simulink model "Grid_Connected_Solar_PV_Array"  (R2023b)
settings: Solver=VariableStepAuto  StartTime=0.0  StopTime=0.5  RelTol=1e-3
undefined symbols (not defined in the file): Ts_Control, Ts_Power
libraries: spsSeriesRLCBranchLib x5, slpidlib x2, spsVoltageMeasurementLib x2, spsACVoltageSourceLib x1, spsCurrentMeasurementLib x1, spsPVArrayLib x1, spsPWMGenerator2LevelLib x1, spsSeriesRLCLoadLib x1, spsFundamentalPLLDrivenLib x1, spsMeanLib x1, spsPLLLib x1, spsAlphaBetaZerotodq0Lib x1
settings Model: Creator=HP  LastModifiedBy=HP
settings DataIOCC: SaveOutput=off  SaveState=on  SignalLogging=off  DSMLogging=off  ReturnWorkspaceOutputs=off  LoggingToFile=on

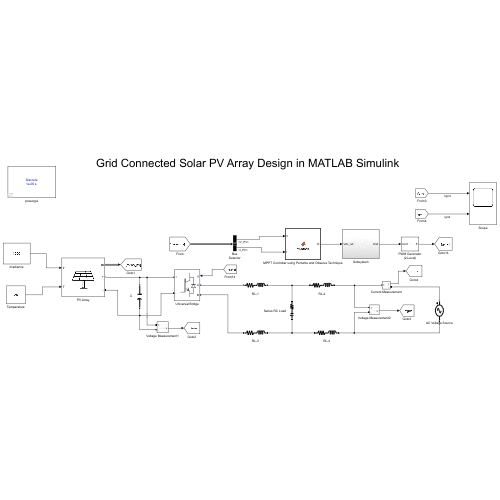
[thumbnail: Simulink's stored preview of the top-level diagram]
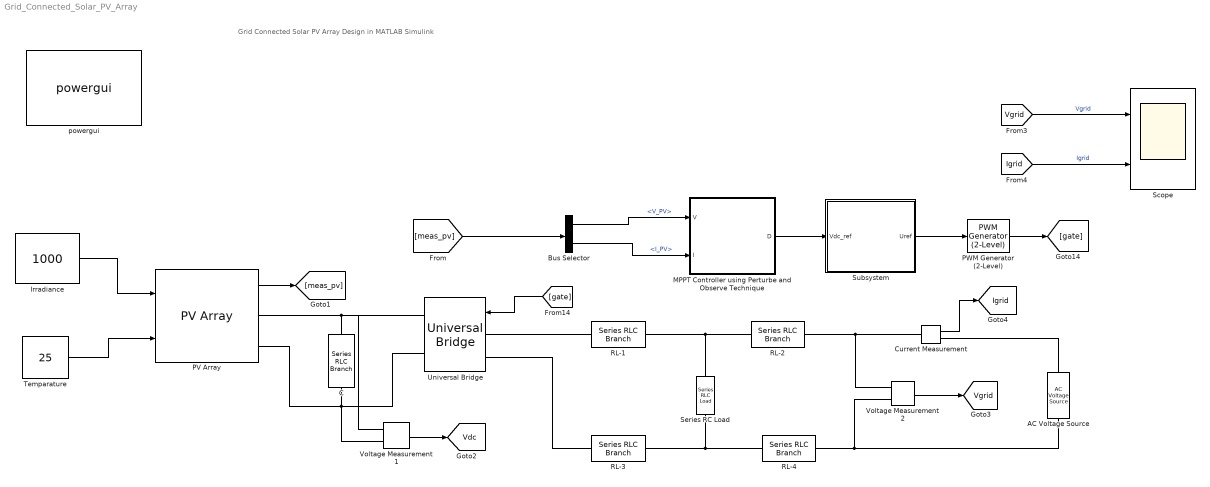
== system Grid_Connected_Solar_PV_Array ==
  note: Grid Connected Solar PV Array Design in MATLAB Simulink
  AC Voltage Source : spsACVoltageSourceLib/AC Voltage Source  Amplitude=240*sqrt(2)  Phase=0  Frequency=50  SampleTime=0  Measurements=None  BusType=swing  Pref=10e3  Qref=0  Qmin=-inf  Qmax=+inf
  Bus Selector : BusSelector  OutputSignals=V_PV,I_PV
  C : spsSeriesRLCBranchLib/Series RLC Branch  LConnTagsString=__new0  RConnTagsString=__new0  BranchType=C  Resistance=1  Inductance=1e-3  SetiL0=off  InitialCurrent=0  Capacitance=3000e-6  Setx0=on  InitialVoltage=420  Measurements=None
  Current Measurement : spsCurrentMeasurementLib/Current Measurement  PhasorSimulation=off  OutputType=Complex  PSBequivalent=0
  Irradiance : Constant  Value=1000
  MPPT Controller using Perturbe and Observe Technique : MATLAB Function  TreatAsAtomicUnit=on
  PV Array : spsPVArrayLib/PV Array  Npar=1  Nser=14  PlotType=array @ 1000 W/m2 & specified temperatures  S_vec="[ 1000  500  100 ]"  Temp_C_vec="[ 45 25  ]"  ModuleName=A10Green Technology A10J-M60-240  PlotWhenSelected=off  Pm=240.5376  Ncell=60  Voc=36.84  Isc=8.32  Vm=30.72  Im=7.83  beta_Voc_pc=-0.359  alpha_Isc_pc=0.096995  beta_Voc=-0.13226  alpha_Isc=0.00807  IL=8.3299  I0=2.8736e-10  nI=0.99259  Rsh=330.6558  Rs=0.19366  RobustModel=off  RobustCellTemperature=313.3991  BAL=on  Tc=1e-6  Tfilter=5e-5
  PWM Generator (2-Level) : spsPWMGenerator2LevelLib/PWM Generator (2-Level)  ModulatorType=Single-phase full-bridge (4 pulses)  ModulatorMode=Unsynchronized  Fc=5e3  Pc=90  nF=27  MinMax="[ -1  1 ]"  SamplingTechnique=Natural  ModulatingSignals=off  m=0.8  Freq=60  Phase=0  Ts=Ts_Power  ShowCarrierOutport=off
  RL-{1..4} (4 alike) : spsSeriesRLCBranchLib/Series RLC Branch  LConnTagsString=__new0  RConnTagsString=__new0  BranchType=RL  Resistance=8.2e-3  Inductance=2.18e-3  SetiL0=off  InitialCurrent=0  Capacitance=3000e-6  Setx0=on  InitialVoltage=420  Measurements=None
  Scope : Scope  NumInputPorts=2
  Series RC Load : spsSeriesRLCLoadLib/Series RLC Load  LConnTagsString=a  RConnTagsString=__new0  NominalVoltage=240  NominalFrequency=60  ActivePower=10  InductivePower=0  CapacitivePower=500  Setx0=off  InitialVoltage=0  SetiL0=off  InitialCurrent=0  Measurements=None  LoadType=constant Z
  Subsystem : Subsystem
  Temparature : Constant  Value=25
  Universal Bridge : spsUniversalBridgeLib/Universal Bridge  Arms=2  SnubberResistance=1e5  SnubberCapacitance=inf  Device=IGBT / Diodes  Ron=1e-3  Lon=0  ForwardVoltages="[  0  0  ]"  ForwardVoltage=0  GTOparameters=[ 10e-6 , 20e-6 ]  IGBTparameters=[ 1e-6 , 2e-6 ]  Measurements=None  Measurements_2=None  converterType=Rectifier
  Voltage Measurement1 : spsVoltageMeasurementLib/Voltage Measurement  PhasorSimulation=off  OutputType=Complex  PSBequivalent=0
  Voltage Measurement2 : spsVoltageMeasurementLib/Voltage Measurement  PhasorSimulation=off  OutputType=Complex  PSBequivalent=0
  powergui : sps_lib/powergui  Priority=1  SimulationMode=Discrete  SampleTime=Ts_Power  frequency=60  Iterations=50  frequencyindice=50  Pbase=100e6  ErrMax=1e-4  UnitsV=kV  UnitsW=MW  buscounter=0  FunctionMessages=off  echomessages=off  EnableUseOfTLC=off  CurrentSourceSwitches=off  DisableSnubberDevices=off  DisableRonSwitches=off  DisableVfSwitches=off  DisplayEquations=off  AutomaticDiscreteSolvers=off  SolverType=Tustin/Backward Euler (TBE)  Interpol=off  ExternalGateDelay=off  methode=off  Ts=100  x0status=blocks  SPID=on  SwTol=0  HookPort=off  NonlinearTolerance=1e-4  nMaxIteration=100  ContinueOnMaxIteration=off  RestoreLinks=warning  ResistiveCurrentMeasurement=off  Frange=[0:2:500]  Ylog=off  Xlog=on  ShowGrid=off  save=off  variable=ZData  structure=0  ZoomFFT=off  StartTime=0.0  cycles=1  DisplayStyle=1  fundamental=60  FreqAxis=off  MaxFrequency=1000  frequencyindicesteady=1  RmsSteady=1  display=off
  tag scope: Igrid=global, Vdc=global, Vgrid=global
  wires:
  Temparature/1 -> PV Array/2
  PV Array/1 -> [meas_pv]
  Voltage Measurement1/1 -> [Vdc]
  Voltage Measurement2/1 -> [Vgrid]
  Current Measurement/1 -> [Igrid]
  [meas_pv] -> Bus Selector/1
  Bus Selector/1 -> MPPT Controller using Perturbe and Observe Technique/1(V)  "<V_PV>"
  Bus Selector/2 -> MPPT Controller using Perturbe and Observe Technique/2(I)  "<I_PV>"
  MPPT Controller using Perturbe and Observe Technique/1(D) -> Subsystem/1(Vdc_ref)
  Subsystem/1(Uref) -> PWM Generator (2-Level)/1
  PWM Generator (2-Level)/1 -> [gate]
  [gate] -> Universal Bridge/1
  [Vgrid] -> Scope/1  "Vgrid"
  [Igrid] -> Scope/2  "Igrid"
  Irradiance/1 -> PV Array/1
  connections:
  PV Array/RConn1 -- Universal Bridge/RConn1 -- Voltage Measurement1/LConn1 -- C/LConn1
  PV Array/RConn2 -- C/RConn1 -- Universal Bridge/RConn2 -- Voltage Measurement1/LConn2
  Universal Bridge/LConn1 -- RL-1/LConn1
  RL-3/LConn1 -- Universal Bridge/LConn2
  RL-2/LConn1 -- Series RC Load/LConn1 -- RL-1/RConn1
  RL-3/RConn1 -- RL-4/LConn1 -- Series RC Load/RConn1
  RL-2/RConn1 -- Current Measurement/LConn1 -- Voltage Measurement2/LConn1
  RL-4/RConn1 -- AC Voltage Source/LConn1 -- Voltage Measurement2/LConn2
  AC Voltage Source/RConn1 -- Current Measurement/RConn1

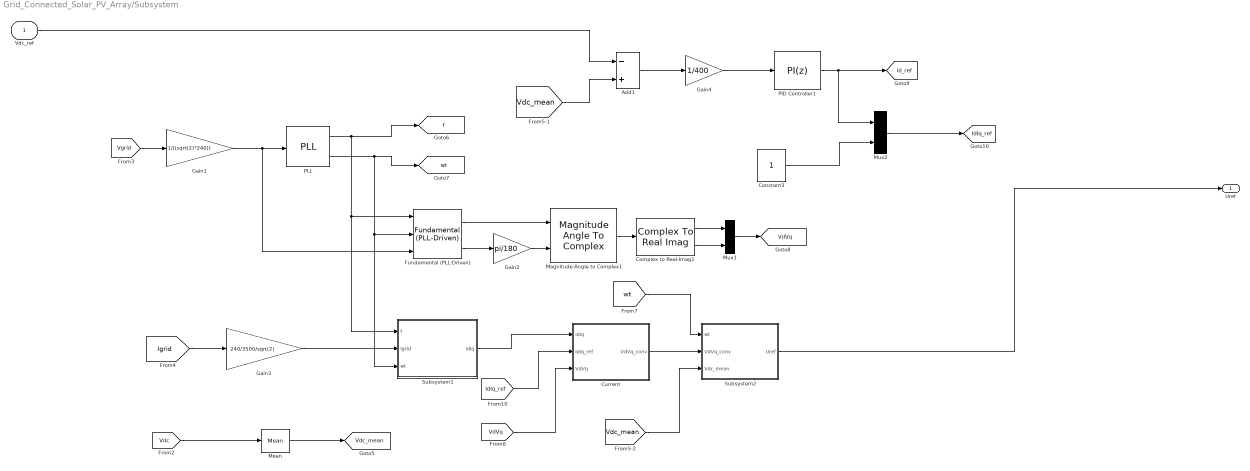
== system Grid_Connected_Solar_PV_Array/Subsystem ==
  Vdc_ref : Inport
  Add1 : Sum  Inputs=-+
  Complex to Real-Imag1 : ComplexToRealImag
  Constant3 : Constant
  Current : Subsystem
  Fundamental (PLL-Driven) : spsFundamentalPLLDrivenLib/Fundamental (PLL-Driven)  Finit=60  Fmin=45  InInit=[1, 0]  Ts=Ts_Control
      settings: LibrarySourceBlock=|
      | sps_lib/Sensors and Measurements/Fundamental
      | (PLL-Driven)
  Gain1 : Gain  Gain=1/((sqrt(2)*240))
  Gain2 : Gain  Gain=pi/180
  Gain3 : Gain  Gain=240/3500/sqrt(2)
  Gain4 : Gain  Gain=1/400
  Magnitude-Angle to Complex1 : MagnitudeAngleToComplex
  Mean : spsMeanLib/Mean  Freq=60  Vinit=420  Ts=Ts_Power
  Mux1 : Mux  Inputs=2
  Mux2 : Mux  Inputs=2
  PID Controller1 : slpidlib/PID Controller  Controller=PI  Form=Parallel  TimeDomain=Discrete-time  UseExternalTs=off  SampleTime=Ts_Control  IntegratorMethod=Forward Euler  FilterMethod=Forward Euler  ControllerParametersSource=internal  P=12  I=200  UseKiTs=off  D=0  N=100  UseFilter=on  TunerSelectOption=Transfer Function Based (PID Tuner App)  InitialConditionSource=internal  InitialConditionForIntegrator=0  InitialConditionForFilter=0  DifferentiatorICPrevScaledInput=0  ExternalReset=none  TrackingMode=off  Kt=1  LimitOutput=off  SatLimitsSource=internal  UpperSaturationLimit=inf  LowerSaturationLimit=-inf  LinearizeAsGain=on  AntiWindupMode=none  Kb=1  LimitIntegrator=off  UpperIntegratorSaturationLimit=inf  LowerIntegratorSaturationLimit=-inf  POutMin=[]  POutMax=[]  IOutMin=[]  IOutMax=[]  DOutMin=[]  DOutMax=[]  NOutMin=[]  NOutMax=[]  SumOutMin=[]  SumOutMax=[]  SaturationOutMin=[]  SaturationOutMax=[]  PParamMin=[]  PParamMax=[]  IParamMin=[]  IParamMax=[]  DParamMin=[]  DParamMax=[]  NParamMin=[]  NParamMax=[]  KbParamMin=[]  KbParamMax=[]  KtParamMin=[]  KtParamMax=[]  KbOutMin=[]  KbOutMax=[]  KtOutMin=[]  KtOutMax=[]  IntegratorOutMin=[]  IntegratorOutMax=[]  FilterOutMin=[]  FilterOutMax=[]  SumI1OutMin=[]  SumI1OutMax=[]  SumI2OutMin=[]  SumI2OutMax=[]  SumI3OutMin=[]  SumI3OutMax=[]  SumI4OutMin=[]  SumI4OutMax=[]  SumDOutMin=[]  SumDOutMax=[]  DifferentiatorOutMin=[]  DifferentiatorOutMax=[]  FilterDiffOutCoefMin=[]  FilterDiffOutCoefMax=[]  ReciprocalOutMin=[]  ReciprocalOutMax=[]  SumDenOutMin=[]  SumDenOutMax=[]  SumNumOutMin=[]  SumNumOutMax=[]  DivideOutMin=[]  DivideOutMax=[]  UdiffTsProdOutMin=[]  UdiffTsProdOutMax=[]  NTsProdOutMin=[]  NTsProdOutMax=[]  UintegralTsProdOutMin=[]  UintegralTsProdOutMax=[]  UngainTsProdOutMin=[]  UngainTsProdOutMax=[]  ClampingZeroOutDataTypeStr=Inherit: Inherit via back propagation  ClampingZeroOutMin=[]  ClampingZeroOutMax=[]  FilterDenConstantOutDataTypeStr=Inherit: Inherit via back propagation  FilterDenConstantOutMin=[]  FilterDenConstantOutMax=[]  PCopyOutDataTypeStr=Inherit: Inherit via back propagation  PCopyOutMin=[]  PCopyOutMax=[]  NCopyOutDataTypeStr=Inherit: Inherit via back propagation  NCopyOutMin=[]  NCopyOutMax=[]  IntegratorContinuousStateAttributes=''  IntegratorStateMustResolveToSignalObject=off  IntegratorRTWStateStorageClass=Auto  FilterContinuousStateAttributes=''  FilterStateMustResolveToSignalObject=off  FilterRTWStateStorageClass=Auto  ParallelPVariant=InternalParameters  IdealPVariant=Disabled  IVariant=InternalParameters  DVariant=Disabled  IntegratorVariant=Discrete  SatVariant=Disabled  AWVariant=Passthrough  PCopyVariant=Disabled  TRVariant=Disabled  FdbkBlocksVariant=Forward  IdealPFdbkVariant=Disabled  SatFdbkVariant=Disabled  DerivativeFilterVariant=Disabled  NVariant=Disabled  NCopyVariant=Disabled_SignalSpec  FilterICVariant=Disabled  IntegratorICVariant=InternalICs  ExternalResetVariant=Disabled  TRSumVariant=Passthrough  SumFdbkVariant=Disabled  SumVariant=Sum_PI  TsampFilterVariant=InternalTs  TsampNgainVariant=Passthrough  TsampIntegralVariant=Disabled_SignalSpec  ExternalSaturationOutDataTypeStr=Inherit: Same as second input
  PLL : spsPLLLib/PLL  Fmin=45  Par_Init=[0, 60]  ParK=[180, 3200, 1]  TcD=1e-4  MaxRateChangeFreq=12  FilterCutOffFreq=25  Ts=0  AGC=on
      settings: LibrarySourceBlock=sps_lib/Control/PLL
  Subsystem1 : Subsystem
  Subsystem2 : Subsystem
  Uref : Outport
  tag scope: IdIq_ref=global, Id_ref=global, VdVq=global, Vdc_mean=global, f=global, wt=global
  wires:
  [Vdc] -> Mean/1
  Mean/1 -> [Vdc_mean]
  Gain1/1 -> PLL/1, Fundamental (PLL-Driven)/3
  [Vgrid] -> Gain1/1
  PLL/1 -> Fundamental (PLL-Driven)/1, Subsystem1/1(f), [f]
  PLL/2 -> [wt], Fundamental (PLL-Driven)/2, Subsystem1/3(wt)
  Fundamental (PLL-Driven)/2 -> Gain2/1
  Fundamental (PLL-Driven)/1 -> Magnitude-Angle to Complex1/1
  Gain2/1 -> Magnitude-Angle to Complex1/2
  Magnitude-Angle to Complex1/1 -> Complex to Real-Imag1/1
  Complex to Real-Imag1/1 -> Mux1/1
  Complex to Real-Imag1/2 -> Mux1/2
  Mux1/1 -> [VdVq]
  [Igrid] -> Gain3/1
  Gain3/1 -> Subsystem1/2(Igrid)
  Vdc_ref/1 -> Add1/1
  [Vdc_mean] -> Add1/2
  Add1/1 -> Gain4/1
  Gain4/1 -> PID Controller1/1
  PID Controller1/1 -> Mux2/1, [Id_ref]
  Constant3/1 -> Mux2/2
  Mux2/1 -> [IdIq_ref]
  [IdIq_ref] -> Current/2(IdIq_ref)
  Subsystem1/1(IdIq) -> Current/1(IdIq)
  [VdVq] -> Current/3(VdVq)
  Current/1(VdVq_conv) -> Subsystem2/2(VdVq_conv)
  [Vdc_mean] -> Subsystem2/3(Vdc_mean)
  [wt] -> Subsystem2/1(wt)
  Subsystem2/1(Uref) -> Uref/1

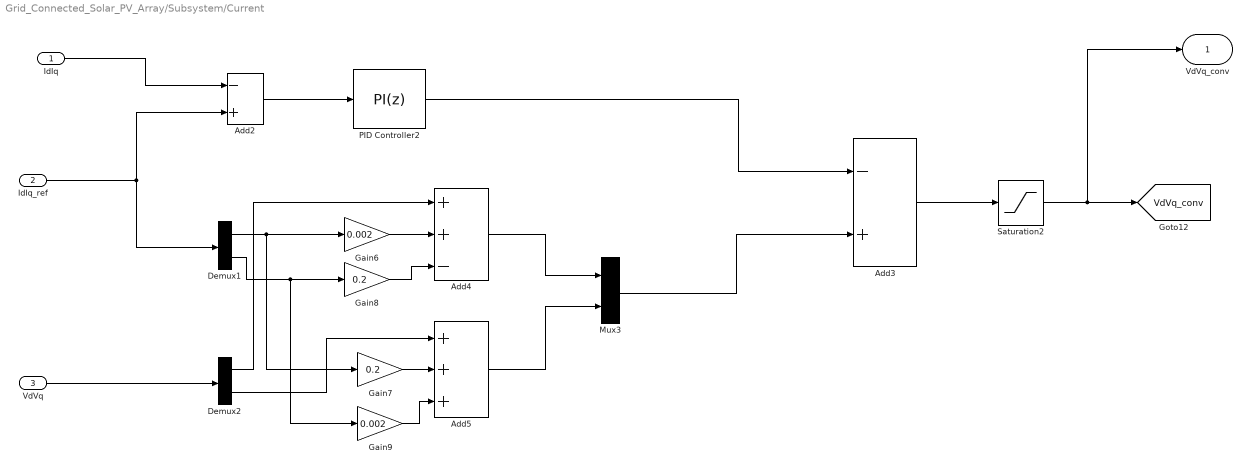
== system Grid_Connected_Solar_PV_Array/Subsystem/Current ==
  IdIq : Inport
  IdIq_ref : Inport  Port=2
  VdVq : Inport  Port=3
  Add2 : Sum  Inputs=-+
  Add3 : Sum  Inputs=-+
  Add4 : Sum  Inputs=++-
  Add5 : Sum  Inputs=+++
  Demux1 : Demux  Outputs=2
  Demux2 : Demux  Outputs=2
  Gain6 : Gain  Gain=0.002
  Gain7 : Gain  Gain=0.2
  Gain8 : Gain  Gain=0.2
  Gain9 : Gain  Gain=0.002
  Mux3 : Mux  Inputs=2
  PID Controller2 : slpidlib/PID Controller  Controller=PI  Form=Parallel  TimeDomain=Discrete-time  UseExternalTs=off  SampleTime=Ts_Control  IntegratorMethod=Forward Euler  FilterMethod=Forward Euler  ControllerParametersSource=internal  P=0.15  I=0.66  UseKiTs=off  D=0  N=100  UseFilter=on  TunerSelectOption=Transfer Function Based (PID Tuner App)  InitialConditionSource=internal  InitialConditionForIntegrator=0  InitialConditionForFilter=0  DifferentiatorICPrevScaledInput=0  ExternalReset=none  TrackingMode=off  Kt=1  LimitOutput=off  SatLimitsSource=internal  UpperSaturationLimit=inf  LowerSaturationLimit=-inf  LinearizeAsGain=on  AntiWindupMode=none  Kb=1  LimitIntegrator=off  UpperIntegratorSaturationLimit=inf  LowerIntegratorSaturationLimit=-inf  POutMin=[]  POutMax=[]  IOutMin=[]  IOutMax=[]  DOutMin=[]  DOutMax=[]  NOutMin=[]  NOutMax=[]  SumOutMin=[]  SumOutMax=[]  SaturationOutMin=[]  SaturationOutMax=[]  PParamMin=[]  PParamMax=[]  IParamMin=[]  IParamMax=[]  DParamMin=[]  DParamMax=[]  NParamMin=[]  NParamMax=[]  KbParamMin=[]  KbParamMax=[]  KtParamMin=[]  KtParamMax=[]  KbOutMin=[]  KbOutMax=[]  KtOutMin=[]  KtOutMax=[]  IntegratorOutMin=[]  IntegratorOutMax=[]  FilterOutMin=[]  FilterOutMax=[]  SumI1OutMin=[]  SumI1OutMax=[]  SumI2OutMin=[]  SumI2OutMax=[]  SumI3OutMin=[]  SumI3OutMax=[]  SumI4OutMin=[]  SumI4OutMax=[]  SumDOutMin=[]  SumDOutMax=[]  DifferentiatorOutMin=[]  DifferentiatorOutMax=[]  FilterDiffOutCoefMin=[]  FilterDiffOutCoefMax=[]  ReciprocalOutMin=[]  ReciprocalOutMax=[]  SumDenOutMin=[]  SumDenOutMax=[]  SumNumOutMin=[]  SumNumOutMax=[]  DivideOutMin=[]  DivideOutMax=[]  UdiffTsProdOutMin=[]  UdiffTsProdOutMax=[]  NTsProdOutMin=[]  NTsProdOutMax=[]  UintegralTsProdOutMin=[]  UintegralTsProdOutMax=[]  UngainTsProdOutMin=[]  UngainTsProdOutMax=[]  ClampingZeroOutDataTypeStr=Inherit: Inherit via back propagation  ClampingZeroOutMin=[]  ClampingZeroOutMax=[]  FilterDenConstantOutDataTypeStr=Inherit: Inherit via back propagation  FilterDenConstantOutMin=[]  FilterDenConstantOutMax=[]  PCopyOutDataTypeStr=Inherit: Inherit via back propagation  PCopyOutMin=[]  PCopyOutMax=[]  NCopyOutDataTypeStr=Inherit: Inherit via back propagation  NCopyOutMin=[]  NCopyOutMax=[]  IntegratorContinuousStateAttributes=''  IntegratorStateMustResolveToSignalObject=off  IntegratorRTWStateStorageClass=Auto  FilterContinuousStateAttributes=''  FilterStateMustResolveToSignalObject=off  FilterRTWStateStorageClass=Auto  ParallelPVariant=InternalParameters  IdealPVariant=Disabled  IVariant=InternalParameters  DVariant=Disabled  IntegratorVariant=Discrete  SatVariant=Disabled  AWVariant=Passthrough  PCopyVariant=Disabled  TRVariant=Disabled  FdbkBlocksVariant=Forward  IdealPFdbkVariant=Disabled  SatFdbkVariant=Disabled  DerivativeFilterVariant=Disabled  NVariant=Disabled  NCopyVariant=Disabled_SignalSpec  FilterICVariant=Disabled  IntegratorICVariant=InternalICs  ExternalResetVariant=Disabled  TRSumVariant=Passthrough  SumFdbkVariant=Disabled  SumVariant=Sum_PI  TsampFilterVariant=InternalTs  TsampNgainVariant=Passthrough  TsampIntegralVariant=Disabled_SignalSpec  ExternalSaturationOutDataTypeStr=Inherit: Same as second input
  Saturation2 : Saturate  UpperLimit=1.5  LowerLimit=-1.5
  VdVq_conv : Outport
  tag scope: VdVq_conv=global
  wires:
  IdIq/1 -> Add2/1
  IdIq_ref/1 -> Demux1/1, Add2/2
  Add2/1 -> PID Controller2/1
  VdVq/1 -> Demux2/1
  Demux2/1 -> Add4/1
  Demux2/2 -> Add5/1
  Gain6/1 -> Add4/2
  Gain7/1 -> Add5/2
  Demux1/1 -> Gain7/1, Gain6/1
  Gain8/1 -> Add4/3
  Demux1/2 -> Gain9/1, Gain8/1
  Gain9/1 -> Add5/3
  Add4/1 -> Mux3/1
  Add5/1 -> Mux3/2
  PID Controller2/1 -> Add3/1
  Mux3/1 -> Add3/2
  Add3/1 -> Saturation2/1
  Saturation2/1 -> VdVq_conv/1, [VdVq_conv]

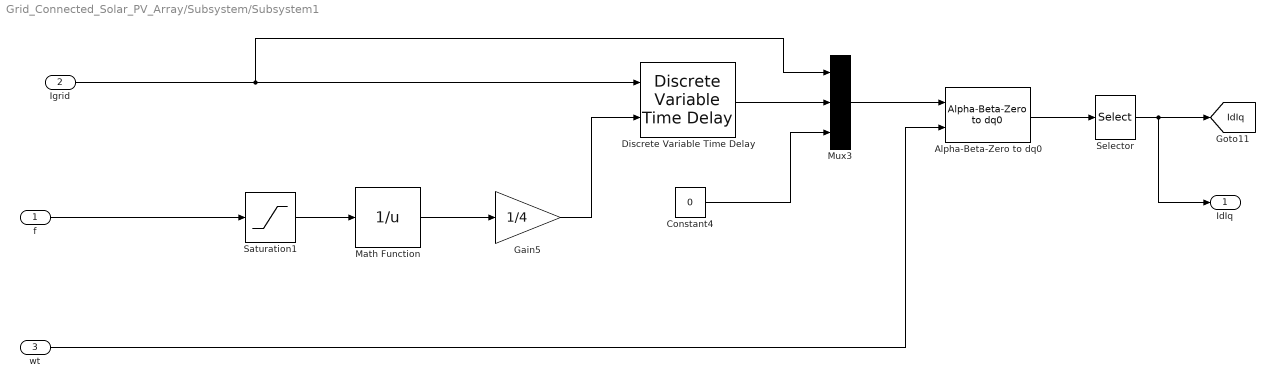
== system Grid_Connected_Solar_PV_Array/Subsystem/Subsystem1 ==
  f : Inport
  Igrid : Inport  Port=2
  wt : Inport  Port=3
  Alpha-Beta-Zero to dq0 : spsAlphaBetaZerotodq0Lib/Alpha-Beta-Zero to dq0  Alignment=90 degrees behind phase A axis
  Constant4 : Constant  Value=0
  Discrete Variable Time Delay : spsDiscreteVariableTimeDelayLib/Discrete Variable Time Delay  MaxDelay=1  InitialValue=0  Ts=Ts_Control  DFT=on
      settings: LibrarySourceBlock=|
      | sps_lib/Control/Discrete Variable
      | Time Delay
  Gain5 : Gain  Gain=1/4
  Math Function : Math  Operator=reciprocal
  Mux3 : Mux  Inputs=3
  Saturation1 : Saturate  UpperLimit=70  LowerLimit=40
  Selector : Selector  InputPortWidth=3  IndexOptions=Index vector (dialog)  Indices=[1 2]  OutputSizes=1
  IdIq : Outport
  tag scope: IdIq=global
  wires:
  f/1 -> Saturation1/1
  Saturation1/1 -> Math Function/1
  Math Function/1 -> Gain5/1
  Gain5/1 -> Discrete Variable Time Delay/2
  Igrid/1 -> Discrete Variable Time Delay/1, Mux3/1
  Discrete Variable Time Delay/1 -> Mux3/2
  Constant4/1 -> Mux3/3
  Mux3/1 -> Alpha-Beta-Zero to dq0/1
  wt/1 -> Alpha-Beta-Zero to dq0/2
  Alpha-Beta-Zero to dq0/1 -> Selector/1
  Selector/1 -> IdIq/1, [IdIq]

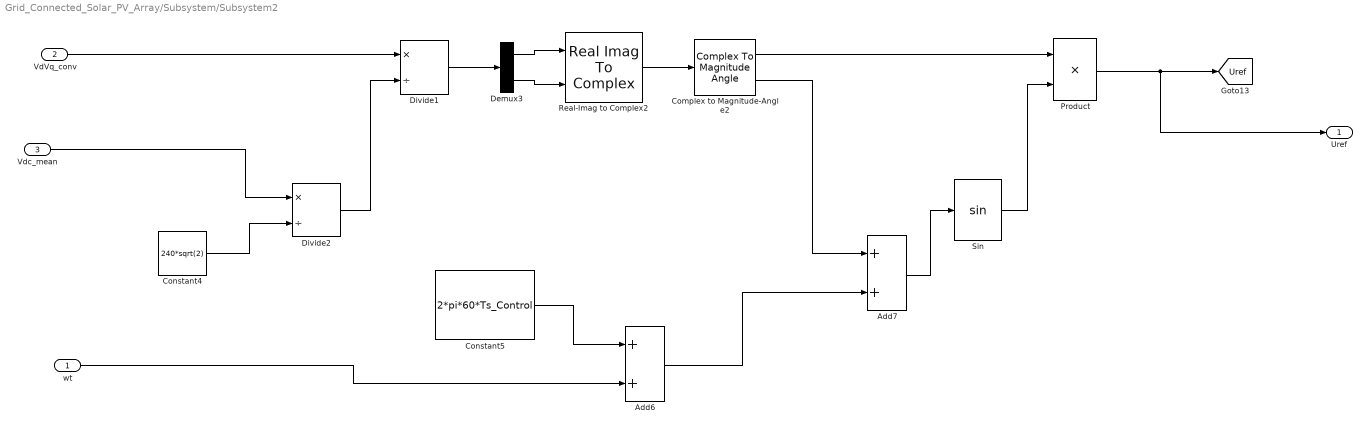
== system Grid_Connected_Solar_PV_Array/Subsystem/Subsystem2 ==
  wt : Inport
  VdVq_conv : Inport  Port=2
  Vdc_mean : Inport  Port=3
  Add6 : Sum
  Add7 : Sum
  Complex to Magnitude-Angle2 : ComplexToMagnitudeAngle
  Constant4 : Constant  Value=240*sqrt(2)
  Constant5 : Constant  Value=2*pi*60*Ts_Control
  Demux3 : Demux  Outputs=2
  Divide1 : Product  Inputs=*/
  Divide2 : Product  Inputs=*/
  Product : Product
  Real-Imag to Complex2 : RealImagToComplex
  Sin : Trigonometry
  Uref : Outport
  tag scope: Uref=global
  wires:
  Vdc_mean/1 -> Divide2/1
  Constant4/1 -> Divide2/2
  VdVq_conv/1 -> Divide1/1
  Divide2/1 -> Divide1/2
  Divide1/1 -> Demux3/1
  Real-Imag to Complex2/1 -> Complex to Magnitude-Angle2/1
  Demux3/1 -> Real-Imag to Complex2/1
  Demux3/2 -> Real-Imag to Complex2/2
  Complex to Magnitude-Angle2/1 -> Product/1
  wt/1 -> Add6/2
  Constant5/1 -> Add6/1
  Add6/1 -> Add7/2
  Complex to Magnitude-Angle2/2 -> Add7/1
  Add7/1 -> Sin/1
  Sin/1 -> Product/2
  Product/1 -> Uref/1, [Uref]

== matlab function Grid_Connected_Solar_PV_Array/MPPT Controller using Perturbe and Observe Technique ==
  data: V input; D output; I input
function D = Muntasir( V, I )
% MPPT controller based on the Perturb & Observe algorithm.
% D output = Reference for DC link voltage (Vdc_ref)
% Enabled input = 1 to enable the MPPT controller
% V input = PV array terminal voltage (V)
% I input = PV array current (A)
% Param input:
Dinit = 425;   % Initial value for Vdc_ref
Dmax  = 450;   % Maximum value for Vdc_ref
Dmin  = 375;   % Minimum value for Vdc_ref
deltaD = 0.003; % Increment value used to increase/decrease Vdc_ref
persistent Vold Pold Dold;
dataType = 'double';
if isempty(Vold)
    Vold = 0;
    Pold = 0;
    Dold = Dinit;
end
P  = V*I;
dV = V - Vold;
dP = P - Pold;

if dP ~= 0
    if dP < 0
        if dV < 0
            D = Dold + deltaD;
        else
            D = Dold - deltaD;
        end
    else
         if dV < 0
            D = Dold - deltaD;
        else
            D = Dold + deltaD;
        end
    end
else
    D = Dold;
end

if D >= Dmax || D <= Dmin
    D = Dold;
end
Dold = D;
Vold = V;
Pold = P;
